simulink model "Simu6_Part2"  (R2023a)
settings: Solver=FixedStepAuto  StartTime=0.0  StopTime=0.1  FixedStep=1e-7  RelTol=1e-3
libraries: spsIGBTDiodeLib x4, spsACVoltageSourceLib x1, spsDCVoltageSourceLib x1, spsSeriesRLCBranchLib x1
settings Model: Creator=DELL  LastModifiedBy=11094
settings DataIOCC: ReturnWorkspaceOutputs=off
settings OptimizationCC: ReuseModelBlockBuffer=off

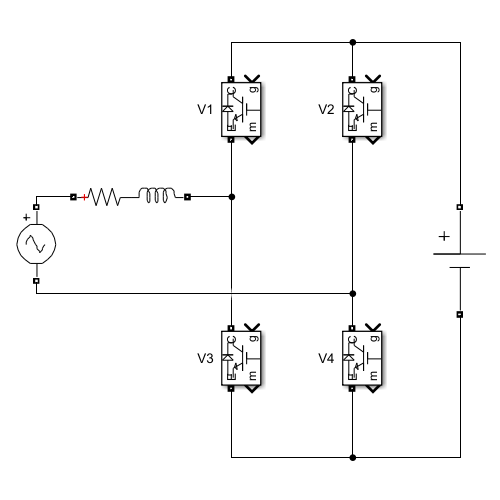
[thumbnail: Simulink's stored preview of the top-level diagram]
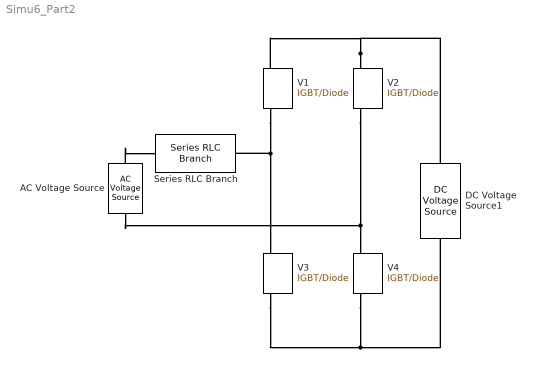
== system Simu6_Part2 ==
  AC Voltage Source : spsACVoltageSourceLib/AC Voltage Source  Amplitude=220*sqrt(2)  Phase=0  Frequency=50  SampleTime=0  Measurements=None  BusType=swing  Pref=10e3  Qref=0  Qmin=-inf  Qmax=+inf
  DC Voltage Source1 : spsDCVoltageSourceLib/DC Voltage Source  Amplitude=570  Measurements=None
  Series RLC Branch : spsSeriesRLCBranchLib/Series RLC Branch  LConnTagsString=__new0  RConnTagsString=__new0  BranchType=RL  Resistance=0  Inductance=4e-3  SetiL0=off  InitialCurrent=0  Capacitance=1e-6  Setx0=off  InitialVoltage=0  Measurements=None
  V{1..4} (4 alike) : spsIGBTDiodeLib/IGBT//Diode  Ron=1e-3  Rs=1e5  Cs=inf  Measurements=on
  connections:
  V2/LConn1 -- DC Voltage Source1/RConn1 -- V1/LConn1
  AC Voltage Source/LConn1 -- V2/RConn1 -- V4/LConn1
  AC Voltage Source/RConn1 -- Series RLC Branch/LConn1
  V1/RConn1 -- V3/LConn1 -- Series RLC Branch/RConn1
  V3/RConn1 -- DC Voltage Source1/LConn1 -- V4/RConn1
